simulink model "factorial2"  (R2018b)
settings: Solver=FixedStepDiscrete  StartTime=0.0  StopTime=10.0  RelTol=1e-3
settings Model: Creator=Romario  LastModifiedBy=Romario
settings OptimizationCC: DefaultParameterBehavior=Inlined  EnhancedBackFolding=on  PassReuseOutputArgsAs=Individual arguments  OptimizeBlockOrder=speed  DifferentSizesBufferReuse=on  OptimizationCustomize=off
settings DebuggingCC: UnderspecifiedInitializationDetection=Classic  MergeDetectMultiDrivingBlocksExec=none  ParameterTunabilityLossMsg=error
settings ModelReferenceCC: PropagateSignalLabelsOutOfModel=off
settings SFSimCC: MATLABDynamicMemAlloc=off
settings RTWCC: SystemTargetFile=ert.tlc  GenCodeOnly=on  TemplateMakefile=ert_default_tmf  GenerateReport=on  IncludeHyperlinkInReport=on  LaunchReport=on  GenerateTraceInfo=on  GenerateTraceReport=on  GenerateTraceReportSl=on  GenerateTraceReportSf=on  GenerateTraceReportEml=on
settings CodeAppCC: ForceParamTrailComments=on  IgnoreCustomStorageClasses=off  OperatorAnnotations=on  SimulinkDataObjDesc=on  SFDataObjDesc=on  InsertBlockDesc=on
settings ERTTargetCC: TargetLangStandard=C99 (ISO)  GenerateSampleERTMain=on  InlinedParameterPlacement=NonHierarchical  ERTCustomFileTemplate=example_file_process.tlc

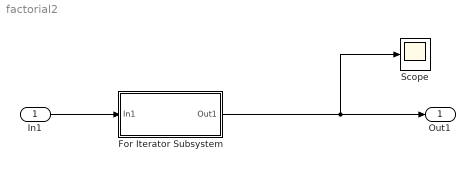
== system factorial2 ==
  In1 : Inport
  For Iterator Subsystem : Subsystem  TreatAsAtomicUnit=on
  Scope : Scope
  Out1 : Outport
  wires:
  In1/1 -> For Iterator Subsystem/1(In1)
  For Iterator Subsystem/1(Out1) -> Scope/1, Out1/1

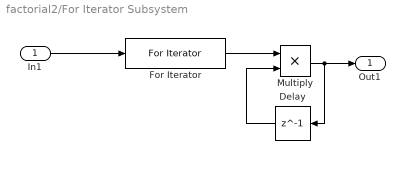
== system factorial2/For Iterator Subsystem ==
  In1 : Inport
  Delay : Delay  DelayLength=1  InitialCondition=1
  For Iterator : ForIterator  IterationSource=external
  Multiply : Product  OutDataTypeStr=int32
  Out1 : Outport
  wires:
  In1/1 -> For Iterator/1
  Multiply/1 -> Out1/1, Delay/1
  Delay/1 -> Multiply/2
  For Iterator/1 -> Multiply/1
